simulink model "IEEE34BARRAS"  (R2018a)
settings: Solver=ode4  StartTime=0.0  StopTime=48*T  FixedStep=Ts  RelTol=1e-3  EnableMultiTasking=on
InitFcn:
  | close
  | clc
  | clear
  | n=2^8;
  | f=60;
  | T=1/f;
  | Ts=1/(f*n);
  | NT=18;
  | set_param('IEEE34BARRAS/EMISOR-RECEPTOR/TCP_IP_RX1/ESCRITURA', 'Value','[0,0,0,0,0,0,0,0,0,0,0,0,0,0,0,0,0,0,0,0,0,0,0,0,0,0,0,0,0,0,0,0,0,0,0,0,0,0,0,0,0]')
  | set_param('IEEE34BARRAS/EMISOR-RECEPTOR/TCP_IP_RX1/RETARDO', 'Value','0')
  | run script_client_1_inicio1.m
undefined symbols (not defined in the file or in its folder): D1, Delta, DiscIntNeverNeededParam, Ip1
libraries: powerlib x313, simulink x15, libreria_medidores1T x3, libreria_comunicaciones_cliente1T x2
(part 2 of 5)

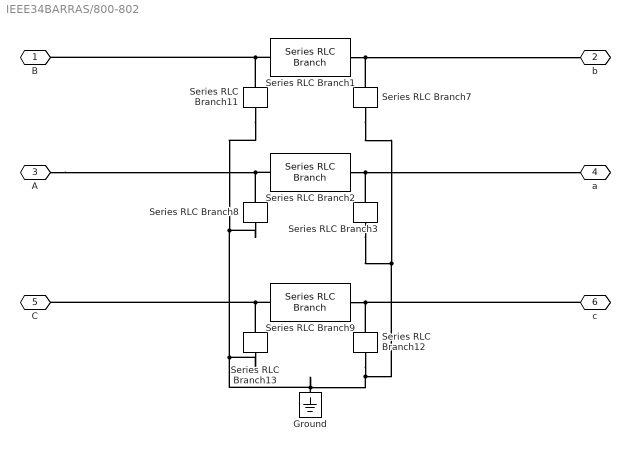
== system IEEE34BARRAS/800-802 ==
  Ground : powerlib/Elements/Ground  LConnTagsString=a
  Series RLC Branch1 : powerlib/Elements/Series RLC Branch  LConnTagsString=__new0  RConnTagsString=__new0  BranchType=RL  Resistance=R(1)*Ft  Inductance=L(1)*Ft  SetiL0=off  InitialCurrent=0  Capacitance=8.4659e-09  Setx0=off  InitialVoltage=0  Measurements=None
  Series RLC Branch11 : powerlib/Elements/Series RLC Branch  LConnTagsString=__new0  RConnTagsString=__new0  BranchType=C  Resistance=0.13252  Inductance=0.0024863  SetiL0=off  InitialCurrent=0  Capacitance=C(1)/2*Ft  Setx0=off  InitialVoltage=0  Measurements=None
  Series RLC Branch12 : powerlib/Elements/Series RLC Branch  LConnTagsString=__new0  RConnTagsString=__new0  BranchType=C  Resistance=0.13252  Inductance=0.0024863  SetiL0=off  InitialCurrent=0  Capacitance=C(3)/2*Ft  Setx0=off  InitialVoltage=0  Measurements=None
  Series RLC Branch13 : powerlib/Elements/Series RLC Branch  LConnTagsString=__new0  RConnTagsString=__new0  BranchType=C  Resistance=0.13252  Inductance=0.0024863  SetiL0=off  InitialCurrent=0  Capacitance=C(3)/2*Ft  Setx0=off  InitialVoltage=0  Measurements=None
  Series RLC Branch2 : powerlib/Elements/Series RLC Branch  LConnTagsString=__new0  RConnTagsString=__new0  BranchType=RL  Resistance=R(2)*Ft  Inductance=L(2)*Ft  SetiL0=off  InitialCurrent=0  Capacitance=8.4659e-09  Setx0=off  InitialVoltage=0  Measurements=None
  Series RLC Branch3 : powerlib/Elements/Series RLC Branch  LConnTagsString=__new0  RConnTagsString=__new0  BranchType=C  Resistance=0.13252  Inductance=0.0024863  SetiL0=off  InitialCurrent=0  Capacitance=C(2)/2*Ft  Setx0=off  InitialVoltage=0  Measurements=None
  Series RLC Branch7 : powerlib/Elements/Series RLC Branch  LConnTagsString=__new0  RConnTagsString=__new0  BranchType=C  Resistance=0.13252  Inductance=0.0024863  SetiL0=off  InitialCurrent=0  Capacitance=C(1)/2*Ft  Setx0=off  InitialVoltage=0  Measurements=None
  Series RLC Branch8 : powerlib/Elements/Series RLC Branch  LConnTagsString=__new0  RConnTagsString=__new0  BranchType=C  Resistance=0.13252  Inductance=0.0024863  SetiL0=off  InitialCurrent=0  Capacitance=C(2)/2*Ft  Setx0=off  InitialVoltage=0  Measurements=None
  Series RLC Branch9 : powerlib/Elements/Series RLC Branch  LConnTagsString=__new0  RConnTagsString=__new0  BranchType=RL  Resistance=R(3)*Ft  Inductance=L(3)*Ft  SetiL0=off  InitialCurrent=0  Capacitance=8.4659e-09  Setx0=off  InitialVoltage=0  Measurements=None
  B : PMIOPort  Side=Left
  b : PMIOPort  Port=2  Side=Right
  A : PMIOPort  Port=3  Side=Left
  a : PMIOPort  Port=4  Side=Right
  C : PMIOPort  Port=5  Side=Left
  c : PMIOPort  Port=6  Side=Right
  connections:
  Series RLC Branch11/LConn1 -- Series RLC Branch1/LConn1 -- B/RConn1
  Series RLC Branch1/RConn1 -- Series RLC Branch7/LConn1 -- b/RConn1
  Ground/LConn1 -- Series RLC Branch8/RConn1 -- Series RLC Branch11/RConn1 -- Series RLC Branch13/RConn1 -- Series RLC Branch7/RConn1 -- Series RLC Branch3/RConn1 -- Series RLC Branch12/RConn1
  Series RLC Branch8/LConn1 -- A/RConn1 -- Series RLC Branch2/LConn1
  Series RLC Branch3/LConn1 -- a/RConn1 -- Series RLC Branch2/RConn1
  Series RLC Branch9/LConn1 -- C/RConn1 -- Series RLC Branch13/LConn1
  Series RLC Branch9/RConn1 -- c/RConn1 -- Series RLC Branch12/LConn1

== system IEEE34BARRAS/802-806 ==
  Ground : powerlib/Elements/Ground  LConnTagsString=a
  Series RLC Branch1 : powerlib/Elements/Series RLC Branch  LConnTagsString=__new0  RConnTagsString=__new0  BranchType=RL  Resistance=R(1)*Ft  Inductance=L(1)*Ft  SetiL0=off  InitialCurrent=0  Capacitance=8.4659e-09  Setx0=off  InitialVoltage=0  Measurements=None
  Series RLC Branch11 : powerlib/Elements/Series RLC Branch  LConnTagsString=__new0  RConnTagsString=__new0  BranchType=C  Resistance=0.13252  Inductance=0.0024863  SetiL0=off  InitialCurrent=0  Capacitance=C(1)/2*Ft  Setx0=off  InitialVoltage=0  Measurements=None
  Series RLC Branch12 : powerlib/Elements/Series RLC Branch  LConnTagsString=__new0  RConnTagsString=__new0  BranchType=C  Resistance=0.13252  Inductance=0.0024863  SetiL0=off  InitialCurrent=0  Capacitance=C(3)/2*Ft  Setx0=off  InitialVoltage=0  Measurements=None
  Series RLC Branch13 : powerlib/Elements/Series RLC Branch  LConnTagsString=__new0  RConnTagsString=__new0  BranchType=C  Resistance=0.13252  Inductance=0.0024863  SetiL0=off  InitialCurrent=0  Capacitance=C(3)/2*Ft  Setx0=off  InitialVoltage=0  Measurements=None
  Series RLC Branch2 : powerlib/Elements/Series RLC Branch  LConnTagsString=__new0  RConnTagsString=__new0  BranchType=RL  Resistance=R(2)*Ft  Inductance=L(2)*Ft  SetiL0=off  InitialCurrent=0  Capacitance=8.4659e-09  Setx0=off  InitialVoltage=0  Measurements=None
  Series RLC Branch3 : powerlib/Elements/Series RLC Branch  LConnTagsString=__new0  RConnTagsString=__new0  BranchType=C  Resistance=0.13252  Inductance=0.0024863  SetiL0=off  InitialCurrent=0  Capacitance=C(2)/2*Ft  Setx0=off  InitialVoltage=0  Measurements=None
  Series RLC Branch7 : powerlib/Elements/Series RLC Branch  LConnTagsString=__new0  RConnTagsString=__new0  BranchType=C  Resistance=0.13252  Inductance=0.0024863  SetiL0=off  InitialCurrent=0  Capacitance=C(1)/2*Ft  Setx0=off  InitialVoltage=0  Measurements=None
  Series RLC Branch8 : powerlib/Elements/Series RLC Branch  LConnTagsString=__new0  RConnTagsString=__new0  BranchType=C  Resistance=0.13252  Inductance=0.0024863  SetiL0=off  InitialCurrent=0  Capacitance=C(2)/2*Ft  Setx0=off  InitialVoltage=0  Measurements=None
  Series RLC Branch9 : powerlib/Elements/Series RLC Branch  LConnTagsString=__new0  RConnTagsString=__new0  BranchType=RL  Resistance=R(3)*Ft  Inductance=L(3)*Ft  SetiL0=off  InitialCurrent=0  Capacitance=8.4659e-09  Setx0=off  InitialVoltage=0  Measurements=None
  B : PMIOPort  Side=Left
  b : PMIOPort  Port=2  Side=Right
  A : PMIOPort  Port=3  Side=Left
  a : PMIOPort  Port=4  Side=Right
  C : PMIOPort  Port=5  Side=Left
  c : PMIOPort  Port=6  Side=Right
  connections:
  c/RConn1 -- Series RLC Branch9/RConn1 -- Series RLC Branch12/LConn1
  C/RConn1 -- Series RLC Branch9/LConn1 -- Series RLC Branch13/LConn1
  a/RConn1 -- Series RLC Branch3/LConn1 -- Series RLC Branch2/RConn1
  A/RConn1 -- Series RLC Branch8/LConn1 -- Series RLC Branch2/LConn1
  Series RLC Branch7/RConn1 -- Series RLC Branch13/RConn1 -- Series RLC Branch11/RConn1 -- Series RLC Branch8/RConn1 -- Ground/LConn1 -- Series RLC Branch12/RConn1 -- Series RLC Branch3/RConn1
  b/RConn1 -- Series RLC Branch1/RConn1 -- Series RLC Branch7/LConn1
  B/RConn1 -- Series RLC Branch1/LConn1 -- Series RLC Branch11/LConn1

== system IEEE34BARRAS/806-808 ==
  Ground : powerlib/Elements/Ground  LConnTagsString=a
  Series RLC Branch1 : powerlib/Elements/Series RLC Branch  LConnTagsString=__new0  RConnTagsString=__new0  BranchType=RL  Resistance=R(1)*Ft  Inductance=L(1)*Ft  SetiL0=off  InitialCurrent=0  Capacitance=8.4659e-09  Setx0=off  InitialVoltage=0  Measurements=None
  Series RLC Branch11 : powerlib/Elements/Series RLC Branch  LConnTagsString=__new0  RConnTagsString=__new0  BranchType=C  Resistance=0.13252  Inductance=0.0024863  SetiL0=off  InitialCurrent=0  Capacitance=C(1)/2*Ft  Setx0=off  InitialVoltage=0  Measurements=None
  Series RLC Branch12 : powerlib/Elements/Series RLC Branch  LConnTagsString=__new0  RConnTagsString=__new0  BranchType=C  Resistance=0.13252  Inductance=0.0024863  SetiL0=off  InitialCurrent=0  Capacitance=C(3)/2*Ft  Setx0=off  InitialVoltage=0  Measurements=None
  Series RLC Branch13 : powerlib/Elements/Series RLC Branch  LConnTagsString=__new0  RConnTagsString=__new0  BranchType=C  Resistance=0.13252  Inductance=0.0024863  SetiL0=off  InitialCurrent=0  Capacitance=C(3)/2*Ft  Setx0=off  InitialVoltage=0  Measurements=None
  Series RLC Branch2 : powerlib/Elements/Series RLC Branch  LConnTagsString=__new0  RConnTagsString=__new0  BranchType=RL  Resistance=R(2)*Ft  Inductance=L(2)*Ft  SetiL0=off  InitialCurrent=0  Capacitance=8.4659e-09  Setx0=off  InitialVoltage=0  Measurements=None
  Series RLC Branch3 : powerlib/Elements/Series RLC Branch  LConnTagsString=__new0  RConnTagsString=__new0  BranchType=C  Resistance=0.13252  Inductance=0.0024863  SetiL0=off  InitialCurrent=0  Capacitance=C(2)/2*Ft  Setx0=off  InitialVoltage=0  Measurements=None
  Series RLC Branch7 : powerlib/Elements/Series RLC Branch  LConnTagsString=__new0  RConnTagsString=__new0  BranchType=C  Resistance=0.13252  Inductance=0.0024863  SetiL0=off  InitialCurrent=0  Capacitance=C(1)/2*Ft  Setx0=off  InitialVoltage=0  Measurements=None
  Series RLC Branch8 : powerlib/Elements/Series RLC Branch  LConnTagsString=__new0  RConnTagsString=__new0  BranchType=C  Resistance=0.13252  Inductance=0.0024863  SetiL0=off  InitialCurrent=0  Capacitance=C(2)/2*Ft  Setx0=off  InitialVoltage=0  Measurements=None
  Series RLC Branch9 : powerlib/Elements/Series RLC Branch  LConnTagsString=__new0  RConnTagsString=__new0  BranchType=RL  Resistance=R(3)*Ft  Inductance=L(3)*Ft  SetiL0=off  InitialCurrent=0  Capacitance=8.4659e-09  Setx0=off  InitialVoltage=0  Measurements=None
  B : PMIOPort  Side=Left
  b : PMIOPort  Port=2  Side=Right
  A : PMIOPort  Port=3  Side=Left
  a : PMIOPort  Port=4  Side=Right
  C : PMIOPort  Port=5  Side=Left
  c : PMIOPort  Port=6  Side=Right
  connections:
  B/RConn1 -- Series RLC Branch11/LConn1 -- Series RLC Branch1/LConn1
  b/RConn1 -- Series RLC Branch7/LConn1 -- Series RLC Branch1/RConn1
  Series RLC Branch8/RConn1 -- Series RLC Branch11/RConn1 -- Series RLC Branch13/RConn1 -- Series RLC Branch3/RConn1 -- Series RLC Branch7/RConn1 -- Series RLC Branch12/RConn1 -- Ground/LConn1
  Series RLC Branch2/LConn1 -- A/RConn1 -- Series RLC Branch8/LConn1
  a/RConn1 -- Series RLC Branch2/RConn1 -- Series RLC Branch3/LConn1
  C/RConn1 -- Series RLC Branch13/LConn1 -- Series RLC Branch9/LConn1
  Series RLC Branch12/LConn1 -- c/RConn1 -- Series RLC Branch9/RConn1

== system IEEE34BARRAS/808-812 ==
  Ground : powerlib/Elements/Ground  LConnTagsString=a
  Series RLC Branch1 : powerlib/Elements/Series RLC Branch  LConnTagsString=__new0  RConnTagsString=__new0  BranchType=RL  Resistance=R(1)*Ft  Inductance=L(1)*Ft  SetiL0=off  InitialCurrent=0  Capacitance=8.4659e-09  Setx0=off  InitialVoltage=0  Measurements=None
  Series RLC Branch11 : powerlib/Elements/Series RLC Branch  LConnTagsString=__new0  RConnTagsString=__new0  BranchType=C  Resistance=0.13252  Inductance=0.0024863  SetiL0=off  InitialCurrent=0  Capacitance=C(1)/2*Ft  Setx0=off  InitialVoltage=0  Measurements=None
  Series RLC Branch12 : powerlib/Elements/Series RLC Branch  LConnTagsString=__new0  RConnTagsString=__new0  BranchType=C  Resistance=0.13252  Inductance=0.0024863  SetiL0=off  InitialCurrent=0  Capacitance=C(3)/2*Ft  Setx0=off  InitialVoltage=0  Measurements=None
  Series RLC Branch13 : powerlib/Elements/Series RLC Branch  LConnTagsString=__new0  RConnTagsString=__new0  BranchType=C  Resistance=0.13252  Inductance=0.0024863  SetiL0=off  InitialCurrent=0  Capacitance=C(3)/2*Ft  Setx0=off  InitialVoltage=0  Measurements=None
  Series RLC Branch2 : powerlib/Elements/Series RLC Branch  LConnTagsString=__new0  RConnTagsString=__new0  BranchType=RL  Resistance=R(2)*Ft  Inductance=L(2)*Ft  SetiL0=off  InitialCurrent=0  Capacitance=8.4659e-09  Setx0=off  InitialVoltage=0  Measurements=None
  Series RLC Branch3 : powerlib/Elements/Series RLC Branch  LConnTagsString=__new0  RConnTagsString=__new0  BranchType=C  Resistance=0.13252  Inductance=0.0024863  SetiL0=off  InitialCurrent=0  Capacitance=C(2)/2*Ft  Setx0=off  InitialVoltage=0  Measurements=None
  Series RLC Branch7 : powerlib/Elements/Series RLC Branch  LConnTagsString=__new0  RConnTagsString=__new0  BranchType=C  Resistance=0.13252  Inductance=0.0024863  SetiL0=off  InitialCurrent=0  Capacitance=C(1)/2*Ft  Setx0=off  InitialVoltage=0  Measurements=None
  Series RLC Branch8 : powerlib/Elements/Series RLC Branch  LConnTagsString=__new0  RConnTagsString=__new0  BranchType=C  Resistance=0.13252  Inductance=0.0024863  SetiL0=off  InitialCurrent=0  Capacitance=C(2)/2*Ft  Setx0=off  InitialVoltage=0  Measurements=None
  Series RLC Branch9 : powerlib/Elements/Series RLC Branch  LConnTagsString=__new0  RConnTagsString=__new0  BranchType=RL  Resistance=R(3)*Ft  Inductance=L(3)*Ft  SetiL0=off  InitialCurrent=0  Capacitance=8.4659e-09  Setx0=off  InitialVoltage=0  Measurements=None
  B : PMIOPort  Side=Left
  b : PMIOPort  Port=2  Side=Right
  A : PMIOPort  Port=3  Side=Left
  a : PMIOPort  Port=4  Side=Right
  C : PMIOPort  Port=5  Side=Left
  c : PMIOPort  Port=6  Side=Right
  connections:
  c/RConn1 -- Series RLC Branch9/RConn1 -- Series RLC Branch12/LConn1
  C/RConn1 -- Series RLC Branch9/LConn1 -- Series RLC Branch13/LConn1
  a/RConn1 -- Series RLC Branch3/LConn1 -- Series RLC Branch2/RConn1
  A/RConn1 -- Series RLC Branch8/LConn1 -- Series RLC Branch2/LConn1
  Series RLC Branch7/RConn1 -- Series RLC Branch3/RConn1 -- Series RLC Branch13/RConn1 -- Series RLC Branch11/RConn1 -- Series RLC Branch8/RConn1 -- Ground/LConn1 -- Series RLC Branch12/RConn1
  b/RConn1 -- Series RLC Branch1/RConn1 -- Series RLC Branch7/LConn1
  B/RConn1 -- Series RLC Branch1/LConn1 -- Series RLC Branch11/LConn1

== system IEEE34BARRAS/812-814 ==
  Ground : powerlib/Elements/Ground  LConnTagsString=a
  Series RLC Branch1 : powerlib/Elements/Series RLC Branch  LConnTagsString=__new0  RConnTagsString=__new0  BranchType=RL  Resistance=R(1)*Ft  Inductance=L(1)*Ft  SetiL0=off  InitialCurrent=0  Capacitance=8.4659e-09  Setx0=off  InitialVoltage=0  Measurements=None
  Series RLC Branch11 : powerlib/Elements/Series RLC Branch  LConnTagsString=__new0  RConnTagsString=__new0  BranchType=C  Resistance=0.13252  Inductance=0.0024863  SetiL0=off  InitialCurrent=0  Capacitance=C(1)/2*Ft  Setx0=off  InitialVoltage=0  Measurements=None
  Series RLC Branch12 : powerlib/Elements/Series RLC Branch  LConnTagsString=__new0  RConnTagsString=__new0  BranchType=C  Resistance=0.13252  Inductance=0.0024863  SetiL0=off  InitialCurrent=0  Capacitance=C(3)/2*Ft  Setx0=off  InitialVoltage=0  Measurements=None
  Series RLC Branch13 : powerlib/Elements/Series RLC Branch  LConnTagsString=__new0  RConnTagsString=__new0  BranchType=C  Resistance=0.13252  Inductance=0.0024863  SetiL0=off  InitialCurrent=0  Capacitance=C(3)/2*Ft  Setx0=off  InitialVoltage=0  Measurements=None
  Series RLC Branch2 : powerlib/Elements/Series RLC Branch  LConnTagsString=__new0  RConnTagsString=__new0  BranchType=RL  Resistance=R(2)*Ft  Inductance=L(2)*Ft  SetiL0=off  InitialCurrent=0  Capacitance=8.4659e-09  Setx0=off  InitialVoltage=0  Measurements=None
  Series RLC Branch3 : powerlib/Elements/Series RLC Branch  LConnTagsString=__new0  RConnTagsString=__new0  BranchType=C  Resistance=0.13252  Inductance=0.0024863  SetiL0=off  InitialCurrent=0  Capacitance=C(2)/2*Ft  Setx0=off  InitialVoltage=0  Measurements=None
  Series RLC Branch7 : powerlib/Elements/Series RLC Branch  LConnTagsString=__new0  RConnTagsString=__new0  BranchType=C  Resistance=0.13252  Inductance=0.0024863  SetiL0=off  InitialCurrent=0  Capacitance=C(1)/2*Ft  Setx0=off  InitialVoltage=0  Measurements=None
  Series RLC Branch8 : powerlib/Elements/Series RLC Branch  LConnTagsString=__new0  RConnTagsString=__new0  BranchType=C  Resistance=0.13252  Inductance=0.0024863  SetiL0=off  InitialCurrent=0  Capacitance=C(2)/2*Ft  Setx0=off  InitialVoltage=0  Measurements=None
  Series RLC Branch9 : powerlib/Elements/Series RLC Branch  LConnTagsString=__new0  RConnTagsString=__new0  BranchType=RL  Resistance=R(3)*Ft  Inductance=L(3)*Ft  SetiL0=off  InitialCurrent=0  Capacitance=8.4659e-09  Setx0=off  InitialVoltage=0  Measurements=None
  B : PMIOPort  Side=Left
  b : PMIOPort  Port=2  Side=Right
  A : PMIOPort  Port=3  Side=Left
  a : PMIOPort  Port=4  Side=Right
  C : PMIOPort  Port=5  Side=Left
  c : PMIOPort  Port=6  Side=Right
  connections:
  B/RConn1 -- Series RLC Branch11/LConn1 -- Series RLC Branch1/LConn1
  b/RConn1 -- Series RLC Branch7/LConn1 -- Series RLC Branch1/RConn1
  Series RLC Branch8/RConn1 -- Series RLC Branch11/RConn1 -- Series RLC Branch13/RConn1 -- Series RLC Branch12/RConn1 -- Series RLC Branch3/RConn1 -- Series RLC Branch7/RConn1 -- Ground/LConn1
  Series RLC Branch2/LConn1 -- A/RConn1 -- Series RLC Branch8/LConn1
  a/RConn1 -- Series RLC Branch2/RConn1 -- Series RLC Branch3/LConn1
  C/RConn1 -- Series RLC Branch13/LConn1 -- Series RLC Branch9/LConn1
  Series RLC Branch12/LConn1 -- c/RConn1 -- Series RLC Branch9/RConn1

== system IEEE34BARRAS/814-850 ==
  Ground : powerlib/Elements/Ground  LConnTagsString=a
  Series RLC Branch1 : powerlib/Elements/Series RLC Branch  LConnTagsString=__new0  RConnTagsString=__new0  BranchType=RL  Resistance=R(1)*Ft  Inductance=L(1)*Ft  SetiL0=off  InitialCurrent=0  Capacitance=8.4659e-09  Setx0=off  InitialVoltage=0  Measurements=None
  Series RLC Branch11 : powerlib/Elements/Series RLC Branch  LConnTagsString=__new0  RConnTagsString=__new0  BranchType=C  Resistance=0.13252  Inductance=0.0024863  SetiL0=off  InitialCurrent=0  Capacitance=C(1)/2*Ft  Setx0=off  InitialVoltage=0  Measurements=None
  Series RLC Branch12 : powerlib/Elements/Series RLC Branch  LConnTagsString=__new0  RConnTagsString=__new0  BranchType=C  Resistance=0.13252  Inductance=0.0024863  SetiL0=off  InitialCurrent=0  Capacitance=C(3)/2*Ft  Setx0=off  InitialVoltage=0  Measurements=None
  Series RLC Branch13 : powerlib/Elements/Series RLC Branch  LConnTagsString=__new0  RConnTagsString=__new0  BranchType=C  Resistance=0.13252  Inductance=0.0024863  SetiL0=off  InitialCurrent=0  Capacitance=C(3)/2*Ft  Setx0=off  InitialVoltage=0  Measurements=None
  Series RLC Branch2 : powerlib/Elements/Series RLC Branch  LConnTagsString=__new0  RConnTagsString=__new0  BranchType=RL  Resistance=R(2)*Ft  Inductance=L(2)*Ft  SetiL0=off  InitialCurrent=0  Capacitance=8.4659e-09  Setx0=off  InitialVoltage=0  Measurements=None
  Series RLC Branch3 : powerlib/Elements/Series RLC Branch  LConnTagsString=__new0  RConnTagsString=__new0  BranchType=C  Resistance=0.13252  Inductance=0.0024863  SetiL0=off  InitialCurrent=0  Capacitance=C(2)/2*Ft  Setx0=off  InitialVoltage=0  Measurements=None
  Series RLC Branch7 : powerlib/Elements/Series RLC Branch  LConnTagsString=__new0  RConnTagsString=__new0  BranchType=C  Resistance=0.13252  Inductance=0.0024863  SetiL0=off  InitialCurrent=0  Capacitance=C(1)/2*Ft  Setx0=off  InitialVoltage=0  Measurements=None
  Series RLC Branch8 : powerlib/Elements/Series RLC Branch  LConnTagsString=__new0  RConnTagsString=__new0  BranchType=C  Resistance=0.13252  Inductance=0.0024863  SetiL0=off  InitialCurrent=0  Capacitance=C(2)/2*Ft  Setx0=off  InitialVoltage=0  Measurements=None
  Series RLC Branch9 : powerlib/Elements/Series RLC Branch  LConnTagsString=__new0  RConnTagsString=__new0  BranchType=RL  Resistance=R(3)*Ft  Inductance=L(3)*Ft  SetiL0=off  InitialCurrent=0  Capacitance=8.4659e-09  Setx0=off  InitialVoltage=0  Measurements=None
  B : PMIOPort  Side=Left
  b : PMIOPort  Port=2  Side=Right
  A : PMIOPort  Port=3  Side=Left
  a : PMIOPort  Port=4  Side=Right
  C : PMIOPort  Port=5  Side=Left
  c : PMIOPort  Port=6  Side=Right
  connections:
  c/RConn1 -- Series RLC Branch9/RConn1 -- Series RLC Branch12/LConn1
  C/RConn1 -- Series RLC Branch9/LConn1 -- Series RLC Branch13/LConn1
  a/RConn1 -- Series RLC Branch3/LConn1 -- Series RLC Branch2/RConn1
  A/RConn1 -- Series RLC Branch8/LConn1 -- Series RLC Branch2/LConn1
  Series RLC Branch7/RConn1 -- Series RLC Branch3/RConn1 -- Series RLC Branch12/RConn1 -- Series RLC Branch13/RConn1 -- Series RLC Branch11/RConn1 -- Series RLC Branch8/RConn1 -- Ground/LConn1
  b/RConn1 -- Series RLC Branch1/RConn1 -- Series RLC Branch7/LConn1
  B/RConn1 -- Series RLC Branch1/LConn1 -- Series RLC Branch11/LConn1

== system IEEE34BARRAS/816-824 ==
  Ground : powerlib/Elements/Ground  LConnTagsString=a
  Series RLC Branch1 : powerlib/Elements/Series RLC Branch  LConnTagsString=__new0  RConnTagsString=__new0  BranchType=RL  Resistance=R(1)*Ft  Inductance=L(1)*Ft  SetiL0=off  InitialCurrent=0  Capacitance=8.4659e-09  Setx0=off  InitialVoltage=0  Measurements=None
  Series RLC Branch11 : powerlib/Elements/Series RLC Branch  LConnTagsString=__new0  RConnTagsString=__new0  BranchType=C  Resistance=0.13252  Inductance=0.0024863  SetiL0=off  InitialCurrent=0  Capacitance=C(1)/2*Ft  Setx0=off  InitialVoltage=0  Measurements=None
  Series RLC Branch12 : powerlib/Elements/Series RLC Branch  LConnTagsString=__new0  RConnTagsString=__new0  BranchType=C  Resistance=0.13252  Inductance=0.0024863  SetiL0=off  InitialCurrent=0  Capacitance=C(3)/2*Ft  Setx0=off  InitialVoltage=0  Measurements=None
  Series RLC Branch13 : powerlib/Elements/Series RLC Branch  LConnTagsString=__new0  RConnTagsString=__new0  BranchType=C  Resistance=0.13252  Inductance=0.0024863  SetiL0=off  InitialCurrent=0  Capacitance=C(3)/2*Ft  Setx0=off  InitialVoltage=0  Measurements=None
  Series RLC Branch2 : powerlib/Elements/Series RLC Branch  LConnTagsString=__new0  RConnTagsString=__new0  BranchType=RL  Resistance=R(2)*Ft  Inductance=L(2)*Ft  SetiL0=off  InitialCurrent=0  Capacitance=8.4659e-09  Setx0=off  InitialVoltage=0  Measurements=None
  Series RLC Branch3 : powerlib/Elements/Series RLC Branch  LConnTagsString=__new0  RConnTagsString=__new0  BranchType=C  Resistance=0.13252  Inductance=0.0024863  SetiL0=off  InitialCurrent=0  Capacitance=C(2)/2*Ft  Setx0=off  InitialVoltage=0  Measurements=None
  Series RLC Branch7 : powerlib/Elements/Series RLC Branch  LConnTagsString=__new0  RConnTagsString=__new0  BranchType=C  Resistance=0.13252  Inductance=0.0024863  SetiL0=off  InitialCurrent=0  Capacitance=C(1)/2*Ft  Setx0=off  InitialVoltage=0  Measurements=None
  Series RLC Branch8 : powerlib/Elements/Series RLC Branch  LConnTagsString=__new0  RConnTagsString=__new0  BranchType=C  Resistance=0.13252  Inductance=0.0024863  SetiL0=off  InitialCurrent=0  Capacitance=C(2)/2*Ft  Setx0=off  InitialVoltage=0  Measurements=None
  Series RLC Branch9 : powerlib/Elements/Series RLC Branch  LConnTagsString=__new0  RConnTagsString=__new0  BranchType=RL  Resistance=R(3)*Ft  Inductance=L(3)*Ft  SetiL0=off  InitialCurrent=0  Capacitance=8.4659e-09  Setx0=off  InitialVoltage=0  Measurements=None
  B : PMIOPort  Side=Left
  b : PMIOPort  Port=2  Side=Right
  A : PMIOPort  Port=3  Side=Left
  a : PMIOPort  Port=4  Side=Right
  C : PMIOPort  Port=5  Side=Left
  c : PMIOPort  Port=6  Side=Right
  connections:
  c/RConn1 -- Series RLC Branch9/RConn1 -- Series RLC Branch12/LConn1
  C/RConn1 -- Series RLC Branch9/LConn1 -- Series RLC Branch13/LConn1
  a/RConn1 -- Series RLC Branch3/LConn1 -- Series RLC Branch2/RConn1
  A/RConn1 -- Series RLC Branch8/LConn1 -- Series RLC Branch2/LConn1
  Series RLC Branch7/RConn1 -- Series RLC Branch3/RConn1 -- Series RLC Branch13/RConn1 -- Series RLC Branch11/RConn1 -- Series RLC Branch8/RConn1 -- Ground/LConn1
  b/RConn1 -- Series RLC Branch1/RConn1 -- Series RLC Branch7/LConn1
  B/RConn1 -- Series RLC Branch1/LConn1 -- Series RLC Branch11/LConn1

== system IEEE34BARRAS/824-828 ==
  Ground : powerlib/Elements/Ground  LConnTagsString=a
  Series RLC Branch1 : powerlib/Elements/Series RLC Branch  LConnTagsString=__new0  RConnTagsString=__new0  BranchType=RL  Resistance=R(1)*Ft  Inductance=L(1)*Ft  SetiL0=off  InitialCurrent=0  Capacitance=8.4659e-09  Setx0=off  InitialVoltage=0  Measurements=None
  Series RLC Branch11 : powerlib/Elements/Series RLC Branch  LConnTagsString=__new0  RConnTagsString=__new0  BranchType=C  Resistance=0.13252  Inductance=0.0024863  SetiL0=off  InitialCurrent=0  Capacitance=C(1)/2*Ft  Setx0=off  InitialVoltage=0  Measurements=None
  Series RLC Branch12 : powerlib/Elements/Series RLC Branch  LConnTagsString=__new0  RConnTagsString=__new0  BranchType=C  Resistance=0.13252  Inductance=0.0024863  SetiL0=off  InitialCurrent=0  Capacitance=C(3)/2*Ft  Setx0=off  InitialVoltage=0  Measurements=None
  Series RLC Branch13 : powerlib/Elements/Series RLC Branch  LConnTagsString=__new0  RConnTagsString=__new0  BranchType=C  Resistance=0.13252  Inductance=0.0024863  SetiL0=off  InitialCurrent=0  Capacitance=C(3)/2*Ft  Setx0=off  InitialVoltage=0  Measurements=None
  Series RLC Branch2 : powerlib/Elements/Series RLC Branch  LConnTagsString=__new0  RConnTagsString=__new0  BranchType=RL  Resistance=R(2)*Ft  Inductance=L(2)*Ft  SetiL0=off  InitialCurrent=0  Capacitance=8.4659e-09  Setx0=off  InitialVoltage=0  Measurements=None
  Series RLC Branch3 : powerlib/Elements/Series RLC Branch  LConnTagsString=__new0  RConnTagsString=__new0  BranchType=C  Resistance=0.13252  Inductance=0.0024863  SetiL0=off  InitialCurrent=0  Capacitance=C(2)/2*Ft  Setx0=off  InitialVoltage=0  Measurements=None
  Series RLC Branch7 : powerlib/Elements/Series RLC Branch  LConnTagsString=__new0  RConnTagsString=__new0  BranchType=C  Resistance=0.13252  Inductance=0.0024863  SetiL0=off  InitialCurrent=0  Capacitance=C(1)/2*Ft  Setx0=off  InitialVoltage=0  Measurements=None
  Series RLC Branch8 : powerlib/Elements/Series RLC Branch  LConnTagsString=__new0  RConnTagsString=__new0  BranchType=C  Resistance=0.13252  Inductance=0.0024863  SetiL0=off  InitialCurrent=0  Capacitance=C(2)/2*Ft  Setx0=off  InitialVoltage=0  Measurements=None
  Series RLC Branch9 : powerlib/Elements/Series RLC Branch  LConnTagsString=__new0  RConnTagsString=__new0  BranchType=RL  Resistance=R(3)*Ft  Inductance=L(3)*Ft  SetiL0=off  InitialCurrent=0  Capacitance=8.4659e-09  Setx0=off  InitialVoltage=0  Measurements=None
  B : PMIOPort  Side=Left
  b : PMIOPort  Port=2  Side=Right
  A : PMIOPort  Port=3  Side=Left
  a : PMIOPort  Port=4  Side=Right
  C : PMIOPort  Port=5  Side=Left
  c : PMIOPort  Port=6  Side=Right
  connections:
  B/RConn1 -- Series RLC Branch11/LConn1 -- Series RLC Branch1/LConn1
  b/RConn1 -- Series RLC Branch7/LConn1 -- Series RLC Branch1/RConn1
  Series RLC Branch8/RConn1 -- Series RLC Branch11/RConn1 -- Series RLC Branch13/RConn1 -- Ground/LConn1 -- Series RLC Branch3/RConn1 -- Series RLC Branch7/RConn1
  Series RLC Branch2/LConn1 -- A/RConn1 -- Series RLC Branch8/LConn1
  a/RConn1 -- Series RLC Branch2/RConn1 -- Series RLC Branch3/LConn1
  C/RConn1 -- Series RLC Branch13/LConn1 -- Series RLC Branch9/LConn1
  Series RLC Branch12/LConn1 -- c/RConn1 -- Series RLC Branch9/RConn1

== system IEEE34BARRAS/828-830 ==
  Ground : powerlib/Elements/Ground  LConnTagsString=a
  Series RLC Branch1 : powerlib/Elements/Series RLC Branch  LConnTagsString=__new0  RConnTagsString=__new0  BranchType=RL  Resistance=R(1)*Ft  Inductance=L(1)*Ft  SetiL0=off  InitialCurrent=0  Capacitance=8.4659e-09  Setx0=off  InitialVoltage=0  Measurements=None
  Series RLC Branch11 : powerlib/Elements/Series RLC Branch  LConnTagsString=__new0  RConnTagsString=__new0  BranchType=C  Resistance=0.13252  Inductance=0.0024863  SetiL0=off  InitialCurrent=0  Capacitance=C(1)/2*Ft  Setx0=off  InitialVoltage=0  Measurements=None
  Series RLC Branch12 : powerlib/Elements/Series RLC Branch  LConnTagsString=__new0  RConnTagsString=__new0  BranchType=C  Resistance=0.13252  Inductance=0.0024863  SetiL0=off  InitialCurrent=0  Capacitance=C(3)/2*Ft  Setx0=off  InitialVoltage=0  Measurements=None
  Series RLC Branch13 : powerlib/Elements/Series RLC Branch  LConnTagsString=__new0  RConnTagsString=__new0  BranchType=C  Resistance=0.13252  Inductance=0.0024863  SetiL0=off  InitialCurrent=0  Capacitance=C(3)/2*Ft  Setx0=off  InitialVoltage=0  Measurements=None
  Series RLC Branch2 : powerlib/Elements/Series RLC Branch  LConnTagsString=__new0  RConnTagsString=__new0  BranchType=RL  Resistance=R(2)*Ft  Inductance=L(2)*Ft  SetiL0=off  InitialCurrent=0  Capacitance=8.4659e-09  Setx0=off  InitialVoltage=0  Measurements=None
  Series RLC Branch3 : powerlib/Elements/Series RLC Branch  LConnTagsString=__new0  RConnTagsString=__new0  BranchType=C  Resistance=0.13252  Inductance=0.0024863  SetiL0=off  InitialCurrent=0  Capacitance=C(2)/2*Ft  Setx0=off  InitialVoltage=0  Measurements=None
  Series RLC Branch7 : powerlib/Elements/Series RLC Branch  LConnTagsString=__new0  RConnTagsString=__new0  BranchType=C  Resistance=0.13252  Inductance=0.0024863  SetiL0=off  InitialCurrent=0  Capacitance=C(1)/2*Ft  Setx0=off  InitialVoltage=0  Measurements=None
  Series RLC Branch8 : powerlib/Elements/Series RLC Branch  LConnTagsString=__new0  RConnTagsString=__new0  BranchType=C  Resistance=0.13252  Inductance=0.0024863  SetiL0=off  InitialCurrent=0  Capacitance=C(2)/2*Ft  Setx0=off  InitialVoltage=0  Measurements=None
  Series RLC Branch9 : powerlib/Elements/Series RLC Branch  LConnTagsString=__new0  RConnTagsString=__new0  BranchType=RL  Resistance=R(3)*Ft  Inductance=L(3)*Ft  SetiL0=off  InitialCurrent=0  Capacitance=8.4659e-09  Setx0=off  InitialVoltage=0  Measurements=None
  B : PMIOPort  Side=Left
  b : PMIOPort  Port=2  Side=Right
  A : PMIOPort  Port=3  Side=Left
  a : PMIOPort  Port=4  Side=Right
  C : PMIOPort  Port=5  Side=Left
  c : PMIOPort  Port=6  Side=Right
  connections:
  c/RConn1 -- Series RLC Branch9/RConn1 -- Series RLC Branch12/LConn1
  C/RConn1 -- Series RLC Branch9/LConn1 -- Series RLC Branch13/LConn1
  a/RConn1 -- Series RLC Branch3/LConn1 -- Series RLC Branch2/RConn1
  A/RConn1 -- Series RLC Branch8/LConn1 -- Series RLC Branch2/LConn1
  Series RLC Branch7/RConn1 -- Series RLC Branch3/RConn1 -- Series RLC Branch13/RConn1 -- Series RLC Branch11/RConn1 -- Series RLC Branch8/RConn1 -- Ground/LConn1 -- Series RLC Branch12/RConn1
  b/RConn1 -- Series RLC Branch1/RConn1 -- Series RLC Branch7/LConn1
  B/RConn1 -- Series RLC Branch1/LConn1 -- Series RLC Branch11/LConn1

== system IEEE34BARRAS/830-854 ==
  Ground : powerlib/Elements/Ground  LConnTagsString=a
  Series RLC Branch1 : powerlib/Elements/Series RLC Branch  LConnTagsString=__new0  RConnTagsString=__new0  BranchType=RL  Resistance=R(1)*Ft  Inductance=L(1)*Ft  SetiL0=off  InitialCurrent=0  Capacitance=8.4659e-09  Setx0=off  InitialVoltage=0  Measurements=None
  Series RLC Branch11 : powerlib/Elements/Series RLC Branch  LConnTagsString=__new0  RConnTagsString=__new0  BranchType=C  Resistance=0.13252  Inductance=0.0024863  SetiL0=off  InitialCurrent=0  Capacitance=C(1)/2*Ft  Setx0=off  InitialVoltage=0  Measurements=None
  Series RLC Branch12 : powerlib/Elements/Series RLC Branch  LConnTagsString=__new0  RConnTagsString=__new0  BranchType=C  Resistance=0.13252  Inductance=0.0024863  SetiL0=off  InitialCurrent=0  Capacitance=C(3)/2*Ft  Setx0=off  InitialVoltage=0  Measurements=None
  Series RLC Branch13 : powerlib/Elements/Series RLC Branch  LConnTagsString=__new0  RConnTagsString=__new0  BranchType=C  Resistance=0.13252  Inductance=0.0024863  SetiL0=off  InitialCurrent=0  Capacitance=C(3)/2*Ft  Setx0=off  InitialVoltage=0  Measurements=None
  Series RLC Branch2 : powerlib/Elements/Series RLC Branch  LConnTagsString=__new0  RConnTagsString=__new0  BranchType=RL  Resistance=R(2)*Ft  Inductance=L(2)*Ft  SetiL0=off  InitialCurrent=0  Capacitance=8.4659e-09  Setx0=off  InitialVoltage=0  Measurements=None
  Series RLC Branch3 : powerlib/Elements/Series RLC Branch  LConnTagsString=__new0  RConnTagsString=__new0  BranchType=C  Resistance=0.13252  Inductance=0.0024863  SetiL0=off  InitialCurrent=0  Capacitance=C(2)/2*Ft  Setx0=off  InitialVoltage=0  Measurements=None
  Series RLC Branch7 : powerlib/Elements/Series RLC Branch  LConnTagsString=__new0  RConnTagsString=__new0  BranchType=C  Resistance=0.13252  Inductance=0.0024863  SetiL0=off  InitialCurrent=0  Capacitance=C(1)/2*Ft  Setx0=off  InitialVoltage=0  Measurements=None
  Series RLC Branch8 : powerlib/Elements/Series RLC Branch  LConnTagsString=__new0  RConnTagsString=__new0  BranchType=C  Resistance=0.13252  Inductance=0.0024863  SetiL0=off  InitialCurrent=0  Capacitance=C(2)/2*Ft  Setx0=off  InitialVoltage=0  Measurements=None
  Series RLC Branch9 : powerlib/Elements/Series RLC Branch  LConnTagsString=__new0  RConnTagsString=__new0  BranchType=RL  Resistance=R(3)*Ft  Inductance=L(3)*Ft  SetiL0=off  InitialCurrent=0  Capacitance=8.4659e-09  Setx0=off  InitialVoltage=0  Measurements=None
  B : PMIOPort  Side=Left
  b : PMIOPort  Port=2  Side=Right
  A : PMIOPort  Port=3  Side=Left
  a : PMIOPort  Port=4  Side=Right
  C : PMIOPort  Port=5  Side=Left
  c : PMIOPort  Port=6  Side=Right
  connections:
  B/RConn1 -- Series RLC Branch11/LConn1 -- Series RLC Branch1/LConn1
  b/RConn1 -- Series RLC Branch7/LConn1 -- Series RLC Branch1/RConn1
  Series RLC Branch8/RConn1 -- Series RLC Branch11/RConn1 -- Series RLC Branch13/RConn1 -- Series RLC Branch12/RConn1 -- Series RLC Branch3/RConn1 -- Series RLC Branch7/RConn1 -- Ground/LConn1
  Series RLC Branch2/LConn1 -- A/RConn1 -- Series RLC Branch8/LConn1
  a/RConn1 -- Series RLC Branch2/RConn1 -- Series RLC Branch3/LConn1
  C/RConn1 -- Series RLC Branch13/LConn1 -- Series RLC Branch9/LConn1
  Series RLC Branch12/LConn1 -- c/RConn1 -- Series RLC Branch9/RConn1

== system IEEE34BARRAS/832-858 ==
  Ground : powerlib/Elements/Ground  LConnTagsString=a
  Series RLC Branch1 : powerlib/Elements/Series RLC Branch  LConnTagsString=__new0  RConnTagsString=__new0  BranchType=RL  Resistance=R(1)*Ft  Inductance=L(1)*Ft  SetiL0=off  InitialCurrent=0  Capacitance=8.4659e-09  Setx0=off  InitialVoltage=0  Measurements=None
  Series RLC Branch11 : powerlib/Elements/Series RLC Branch  LConnTagsString=__new0  RConnTagsString=__new0  BranchType=C  Resistance=0.13252  Inductance=0.0024863  SetiL0=off  InitialCurrent=0  Capacitance=C(1)/2*Ft  Setx0=off  InitialVoltage=0  Measurements=None
  Series RLC Branch12 : powerlib/Elements/Series RLC Branch  LConnTagsString=__new0  RConnTagsString=__new0  BranchType=C  Resistance=0.13252  Inductance=0.0024863  SetiL0=off  InitialCurrent=0  Capacitance=C(3)/2*Ft  Setx0=off  InitialVoltage=0  Measurements=None
  Series RLC Branch13 : powerlib/Elements/Series RLC Branch  LConnTagsString=__new0  RConnTagsString=__new0  BranchType=C  Resistance=0.13252  Inductance=0.0024863  SetiL0=off  InitialCurrent=0  Capacitance=C(3)/2*Ft  Setx0=off  InitialVoltage=0  Measurements=None
  Series RLC Branch2 : powerlib/Elements/Series RLC Branch  LConnTagsString=__new0  RConnTagsString=__new0  BranchType=RL  Resistance=R(2)*Ft  Inductance=L(2)*Ft  SetiL0=off  InitialCurrent=0  Capacitance=8.4659e-09  Setx0=off  InitialVoltage=0  Measurements=None
  Series RLC Branch3 : powerlib/Elements/Series RLC Branch  LConnTagsString=__new0  RConnTagsString=__new0  BranchType=C  Resistance=0.13252  Inductance=0.0024863  SetiL0=off  InitialCurrent=0  Capacitance=C(2)/2*Ft  Setx0=off  InitialVoltage=0  Measurements=None
  Series RLC Branch7 : powerlib/Elements/Series RLC Branch  LConnTagsString=__new0  RConnTagsString=__new0  BranchType=C  Resistance=0.13252  Inductance=0.0024863  SetiL0=off  InitialCurrent=0  Capacitance=C(1)/2*Ft  Setx0=off  InitialVoltage=0  Measurements=None
  Series RLC Branch8 : powerlib/Elements/Series RLC Branch  LConnTagsString=__new0  RConnTagsString=__new0  BranchType=C  Resistance=0.13252  Inductance=0.0024863  SetiL0=off  InitialCurrent=0  Capacitance=C(2)/2*Ft  Setx0=off  InitialVoltage=0  Measurements=None
  Series RLC Branch9 : powerlib/Elements/Series RLC Branch  LConnTagsString=__new0  RConnTagsString=__new0  BranchType=RL  Resistance=R(3)*Ft  Inductance=L(3)*Ft  SetiL0=off  InitialCurrent=0  Capacitance=8.4659e-09  Setx0=off  InitialVoltage=0  Measurements=None
  B : PMIOPort  Side=Left
  b : PMIOPort  Port=2  Side=Right
  A : PMIOPort  Port=3  Side=Left
  a : PMIOPort  Port=4  Side=Right
  C : PMIOPort  Port=5  Side=Left
  c : PMIOPort  Port=6  Side=Right
  connections:
  c/RConn1 -- Series RLC Branch9/RConn1 -- Series RLC Branch12/LConn1
  C/RConn1 -- Series RLC Branch9/LConn1 -- Series RLC Branch13/LConn1
  a/RConn1 -- Series RLC Branch3/LConn1 -- Series RLC Branch2/RConn1
  A/RConn1 -- Series RLC Branch8/LConn1 -- Series RLC Branch2/LConn1
  Series RLC Branch7/RConn1 -- Series RLC Branch3/RConn1 -- Series RLC Branch13/RConn1 -- Series RLC Branch11/RConn1 -- Series RLC Branch8/RConn1 -- Ground/LConn1 -- Series RLC Branch12/RConn1
  b/RConn1 -- Series RLC Branch1/RConn1 -- Series RLC Branch7/LConn1
  B/RConn1 -- Series RLC Branch1/LConn1 -- Series RLC Branch11/LConn1

== system IEEE34BARRAS/834-842 ==
  Ground : powerlib/Elements/Ground  LConnTagsString=a
  Series RLC Branch1 : powerlib/Elements/Series RLC Branch  LConnTagsString=__new0  RConnTagsString=__new0  BranchType=RL  Resistance=R(1)*Ft  Inductance=L(1)*Ft  SetiL0=off  InitialCurrent=0  Capacitance=8.4659e-09  Setx0=off  InitialVoltage=0  Measurements=None
  Series RLC Branch11 : powerlib/Elements/Series RLC Branch  LConnTagsString=__new0  RConnTagsString=__new0  BranchType=C  Resistance=0.13252  Inductance=0.0024863  SetiL0=off  InitialCurrent=0  Capacitance=C(1)/2*Ft  Setx0=off  InitialVoltage=0  Measurements=None
  Series RLC Branch12 : powerlib/Elements/Series RLC Branch  LConnTagsString=__new0  RConnTagsString=__new0  BranchType=C  Resistance=0.13252  Inductance=0.0024863  SetiL0=off  InitialCurrent=0  Capacitance=C(3)/2*Ft  Setx0=off  InitialVoltage=0  Measurements=None
  Series RLC Branch13 : powerlib/Elements/Series RLC Branch  LConnTagsString=__new0  RConnTagsString=__new0  BranchType=C  Resistance=0.13252  Inductance=0.0024863  SetiL0=off  InitialCurrent=0  Capacitance=C(3)/2*Ft  Setx0=off  InitialVoltage=0  Measurements=None
  Series RLC Branch2 : powerlib/Elements/Series RLC Branch  LConnTagsString=__new0  RConnTagsString=__new0  BranchType=RL  Resistance=R(2)*Ft  Inductance=L(2)*Ft  SetiL0=off  InitialCurrent=0  Capacitance=8.4659e-09  Setx0=off  InitialVoltage=0  Measurements=None
  Series RLC Branch3 : powerlib/Elements/Series RLC Branch  LConnTagsString=__new0  RConnTagsString=__new0  BranchType=C  Resistance=0.13252  Inductance=0.0024863  SetiL0=off  InitialCurrent=0  Capacitance=C(2)/2*Ft  Setx0=off  InitialVoltage=0  Measurements=None
  Series RLC Branch7 : powerlib/Elements/Series RLC Branch  LConnTagsString=__new0  RConnTagsString=__new0  BranchType=C  Resistance=0.13252  Inductance=0.0024863  SetiL0=off  InitialCurrent=0  Capacitance=C(1)/2*Ft  Setx0=off  InitialVoltage=0  Measurements=None
  Series RLC Branch8 : powerlib/Elements/Series RLC Branch  LConnTagsString=__new0  RConnTagsString=__new0  BranchType=C  Resistance=0.13252  Inductance=0.0024863  SetiL0=off  InitialCurrent=0  Capacitance=C(2)/2*Ft  Setx0=off  InitialVoltage=0  Measurements=None
  Series RLC Branch9 : powerlib/Elements/Series RLC Branch  LConnTagsString=__new0  RConnTagsString=__new0  BranchType=RL  Resistance=R(3)*Ft  Inductance=L(3)*Ft  SetiL0=off  InitialCurrent=0  Capacitance=8.4659e-09  Setx0=off  InitialVoltage=0  Measurements=None
  B : PMIOPort  Side=Left
  b : PMIOPort  Port=2  Side=Right
  A : PMIOPort  Port=3  Side=Left
  a : PMIOPort  Port=4  Side=Right
  C : PMIOPort  Port=5  Side=Left
  c : PMIOPort  Port=6  Side=Right
  connections:
  c/RConn1 -- Series RLC Branch9/RConn1 -- Series RLC Branch12/LConn1
  C/RConn1 -- Series RLC Branch9/LConn1 -- Series RLC Branch13/LConn1
  a/RConn1 -- Series RLC Branch3/LConn1 -- Series RLC Branch2/RConn1
  A/RConn1 -- Series RLC Branch8/LConn1 -- Series RLC Branch2/LConn1
  Series RLC Branch7/RConn1 -- Series RLC Branch3/RConn1 -- Series RLC Branch13/RConn1 -- Series RLC Branch11/RConn1 -- Series RLC Branch8/RConn1 -- Ground/LConn1 -- Series RLC Branch12/RConn1
  b/RConn1 -- Series RLC Branch1/RConn1 -- Series RLC Branch7/LConn1
  B/RConn1 -- Series RLC Branch1/LConn1 -- Series RLC Branch11/LConn1

== system IEEE34BARRAS/834-860 ==
  Ground : powerlib/Elements/Ground  LConnTagsString=a
  Series RLC Branch1 : powerlib/Elements/Series RLC Branch  LConnTagsString=__new0  RConnTagsString=__new0  BranchType=RL  Resistance=R(1)*Ft  Inductance=L(1)*Ft  SetiL0=off  InitialCurrent=0  Capacitance=8.4659e-09  Setx0=off  InitialVoltage=0  Measurements=None
  Series RLC Branch11 : powerlib/Elements/Series RLC Branch  LConnTagsString=__new0  RConnTagsString=__new0  BranchType=C  Resistance=0.13252  Inductance=0.0024863  SetiL0=off  InitialCurrent=0  Capacitance=C(1)/2*Ft  Setx0=off  InitialVoltage=0  Measurements=None
  Series RLC Branch12 : powerlib/Elements/Series RLC Branch  LConnTagsString=__new0  RConnTagsString=__new0  BranchType=C  Resistance=0.13252  Inductance=0.0024863  SetiL0=off  InitialCurrent=0  Capacitance=C(3)/2*Ft  Setx0=off  InitialVoltage=0  Measurements=None
  Series RLC Branch13 : powerlib/Elements/Series RLC Branch  LConnTagsString=__new0  RConnTagsString=__new0  BranchType=C  Resistance=0.13252  Inductance=0.0024863  SetiL0=off  InitialCurrent=0  Capacitance=C(3)/2*Ft  Setx0=off  InitialVoltage=0  Measurements=None
  Series RLC Branch2 : powerlib/Elements/Series RLC Branch  LConnTagsString=__new0  RConnTagsString=__new0  BranchType=RL  Resistance=R(2)*Ft  Inductance=L(2)*Ft  SetiL0=off  InitialCurrent=0  Capacitance=8.4659e-09  Setx0=off  InitialVoltage=0  Measurements=None
  Series RLC Branch3 : powerlib/Elements/Series RLC Branch  LConnTagsString=__new0  RConnTagsString=__new0  BranchType=C  Resistance=0.13252  Inductance=0.0024863  SetiL0=off  InitialCurrent=0  Capacitance=C(2)/2*Ft  Setx0=off  InitialVoltage=0  Measurements=None
  Series RLC Branch7 : powerlib/Elements/Series RLC Branch  LConnTagsString=__new0  RConnTagsString=__new0  BranchType=C  Resistance=0.13252  Inductance=0.0024863  SetiL0=off  InitialCurrent=0  Capacitance=C(1)/2*Ft  Setx0=off  InitialVoltage=0  Measurements=None
  Series RLC Branch8 : powerlib/Elements/Series RLC Branch  LConnTagsString=__new0  RConnTagsString=__new0  BranchType=C  Resistance=0.13252  Inductance=0.0024863  SetiL0=off  InitialCurrent=0  Capacitance=C(2)/2*Ft  Setx0=off  InitialVoltage=0  Measurements=None
  Series RLC Branch9 : powerlib/Elements/Series RLC Branch  LConnTagsString=__new0  RConnTagsString=__new0  BranchType=RL  Resistance=R(3)*Ft  Inductance=L(3)*Ft  SetiL0=off  InitialCurrent=0  Capacitance=8.4659e-09  Setx0=off  InitialVoltage=0  Measurements=None
  B : PMIOPort  Side=Left
  b : PMIOPort  Port=2  Side=Right
  A : PMIOPort  Port=3  Side=Left
  a : PMIOPort  Port=4  Side=Right
  C : PMIOPort  Port=5  Side=Left
  c : PMIOPort  Port=6  Side=Right
  connections:
  B/RConn1 -- Series RLC Branch11/LConn1 -- Series RLC Branch1/LConn1
  b/RConn1 -- Series RLC Branch7/LConn1 -- Series RLC Branch1/RConn1
  Series RLC Branch8/RConn1 -- Series RLC Branch11/RConn1 -- Series RLC Branch12/RConn1 -- Series RLC Branch3/RConn1 -- Series RLC Branch7/RConn1 -- Ground/LConn1 -- Series RLC Branch13/RConn1
  Series RLC Branch2/LConn1 -- A/RConn1 -- Series RLC Branch8/LConn1
  a/RConn1 -- Series RLC Branch2/RConn1 -- Series RLC Branch3/LConn1
  C/RConn1 -- Series RLC Branch13/LConn1 -- Series RLC Branch9/LConn1
  Series RLC Branch12/LConn1 -- c/RConn1 -- Series RLC Branch9/RConn1

== system IEEE34BARRAS/836-840 ==
  Ground : powerlib/Elements/Ground  LConnTagsString=a
  Series RLC Branch1 : powerlib/Elements/Series RLC Branch  LConnTagsString=__new0  RConnTagsString=__new0  BranchType=RL  Resistance=R(1)*Ft  Inductance=L(1)*Ft  SetiL0=off  InitialCurrent=0  Capacitance=8.4659e-09  Setx0=off  InitialVoltage=0  Measurements=None
  Series RLC Branch11 : powerlib/Elements/Series RLC Branch  LConnTagsString=__new0  RConnTagsString=__new0  BranchType=C  Resistance=0.13252  Inductance=0.0024863  SetiL0=off  InitialCurrent=0  Capacitance=C(1)/2*Ft  Setx0=off  InitialVoltage=0  Measurements=None
  Series RLC Branch12 : powerlib/Elements/Series RLC Branch  LConnTagsString=__new0  RConnTagsString=__new0  BranchType=C  Resistance=0.13252  Inductance=0.0024863  SetiL0=off  InitialCurrent=0  Capacitance=C(3)/2*Ft  Setx0=off  InitialVoltage=0  Measurements=None
  Series RLC Branch13 : powerlib/Elements/Series RLC Branch  LConnTagsString=__new0  RConnTagsString=__new0  BranchType=C  Resistance=0.13252  Inductance=0.0024863  SetiL0=off  InitialCurrent=0  Capacitance=C(3)/2*Ft  Setx0=off  InitialVoltage=0  Measurements=None
  Series RLC Branch2 : powerlib/Elements/Series RLC Branch  LConnTagsString=__new0  RConnTagsString=__new0  BranchType=RL  Resistance=R(2)*Ft  Inductance=L(2)*Ft  SetiL0=off  InitialCurrent=0  Capacitance=8.4659e-09  Setx0=off  InitialVoltage=0  Measurements=None
  Series RLC Branch3 : powerlib/Elements/Series RLC Branch  LConnTagsString=__new0  RConnTagsString=__new0  BranchType=C  Resistance=0.13252  Inductance=0.0024863  SetiL0=off  InitialCurrent=0  Capacitance=C(2)/2*Ft  Setx0=off  InitialVoltage=0  Measurements=None
  Series RLC Branch7 : powerlib/Elements/Series RLC Branch  LConnTagsString=__new0  RConnTagsString=__new0  BranchType=C  Resistance=0.13252  Inductance=0.0024863  SetiL0=off  InitialCurrent=0  Capacitance=C(1)/2*Ft  Setx0=off  InitialVoltage=0  Measurements=None
  Series RLC Branch8 : powerlib/Elements/Series RLC Branch  LConnTagsString=__new0  RConnTagsString=__new0  BranchType=C  Resistance=0.13252  Inductance=0.0024863  SetiL0=off  InitialCurrent=0  Capacitance=C(2)/2*Ft  Setx0=off  InitialVoltage=0  Measurements=None
  Series RLC Branch9 : powerlib/Elements/Series RLC Branch  LConnTagsString=__new0  RConnTagsString=__new0  BranchType=RL  Resistance=R(3)*Ft  Inductance=L(3)*Ft  SetiL0=off  InitialCurrent=0  Capacitance=8.4659e-09  Setx0=off  InitialVoltage=0  Measurements=None
  B : PMIOPort  Side=Left
  b : PMIOPort  Port=2  Side=Right
  A : PMIOPort  Port=3  Side=Left
  a : PMIOPort  Port=4  Side=Right
  C : PMIOPort  Port=5  Side=Left
  c : PMIOPort  Port=6  Side=Right
  connections:
  B/RConn1 -- Series RLC Branch11/LConn1 -- Series RLC Branch1/LConn1
  b/RConn1 -- Series RLC Branch7/LConn1 -- Series RLC Branch1/RConn1
  Series RLC Branch8/RConn1 -- Series RLC Branch11/RConn1 -- Series RLC Branch13/RConn1 -- Series RLC Branch12/RConn1 -- Series RLC Branch3/RConn1 -- Series RLC Branch7/RConn1 -- Ground/LConn1
  Series RLC Branch2/LConn1 -- A/RConn1 -- Series RLC Branch8/LConn1
  a/RConn1 -- Series RLC Branch2/RConn1 -- Series RLC Branch3/LConn1
  C/RConn1 -- Series RLC Branch13/LConn1 -- Series RLC Branch9/LConn1
  Series RLC Branch12/LConn1 -- c/RConn1 -- Series RLC Branch9/RConn1
